simulink model "mymdlcodegenrowmajor"  (R2024b)
settings: Solver=FixedStepAuto  StartTime=0.0  StopTime=10.0  RelTol=1e-3
settings Model: Creator=lyan  LastModifiedBy=lyan
settings OptimizationCC: DefaultParameterBehavior=Inlined  EnhancedBackFolding=on  PassReuseOutputArgsAs=Individual arguments  ZeroExternalMemoryAtStartup=off  ZeroInternalMemoryAtStartup=off  OptimizeBlockOrder=speed  DifferentSizesBufferReuse=on  OptimizationCustomize=off  EfficientTunableParamExpr=on
settings DebuggingCC: ParameterTunabilityLossMsg=error
settings SFSimCC: MATLABDynamicMemAlloc=off
settings RTWCC: Description=Embedded Coder  SystemTargetFile=ert.tlc  TemplateMakefile=ert_default_tmf
settings CodeAppCC: ForceParamTrailComments=on  IgnoreCustomStorageClasses=off  OperatorAnnotations=on  SimulinkDataObjDesc=on  SFDataObjDesc=on  InsertBlockDesc=on
settings ERTTargetCC: TargetLangStandard=C99 (ISO)  GenerateSampleERTMain=on  ArrayLayout=Row-major  ERTCustomFileTemplate=example_file_process.tlc

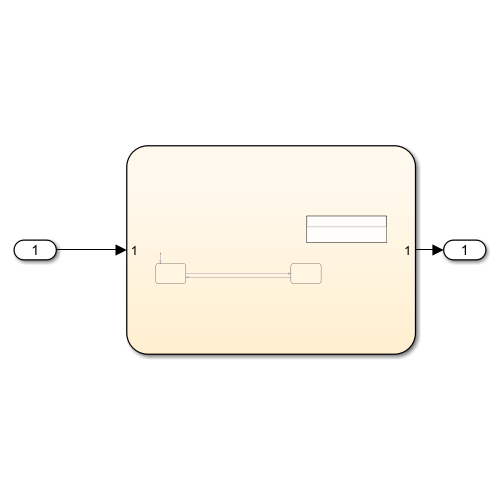
[thumbnail: Simulink's stored preview of the top-level diagram]
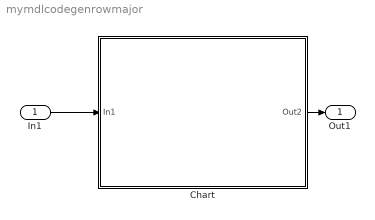
== system mymdlcodegenrowmajor ==
  In1 : Inport
  Chart : Stateflow chart  TreatAsAtomicUnit=on
  Out1 : Outport
  wires:
  In1/1 -> Chart/1(In1)
  Chart/1(Out2) -> Out1/1

== stateflow chart mymdlcodegenrowmajor/Chart ==
  state A
    Out2 = 0;
  state B
    Out2 = 1;
  (default) -> A
  A -> B : [myHasChangedTo(In1,[1,1;1,1])]
  B -> A : [myHasChangedTo(In1,[1,0;0,1])]
  data: u1 function_input; u2 function_input; hasChanged function_output; In1 input; Out2 output
  function hasChanged = myHasChangedTo(u1, u2):
    | function hasChanged = myHasChangedTo(u1, u2)
    | persistent lastStep;
    | if(isempty(lastStep))
    |     lastStep = all(u1(:) == u2(:));
    |     hasChanged = false;
    |     return;
    | end
    | thisStep = all(u1(:) == u2(:));
    | hasChanged = thisStep && xor(thisStep, lastStep);
    | lastStep = thisStep;
    | end
